simulink model "FKtest2"  (Simulink 6.6)
settings: Solver=ode4  StartTime=0.0  StopTime=400  FixedStep=0.05  RelTol=1e-3
values from neighbouring files (symbols this model uses):
  vessel =     [input.mat]    (also in supply.mat)
libraries: marine_gnc x10, simulink x1
(part 1 of 2)
settings Model: Creator=Thor  LastModifiedBy=Thor

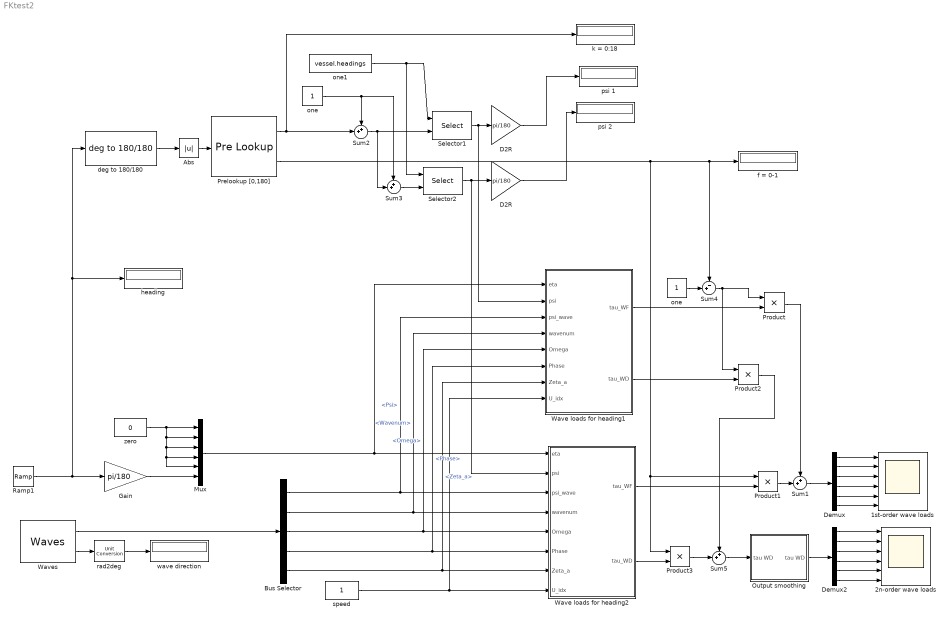
== system FKtest2 ==
  "1st-order wave loads " : Scope  NumInputPorts=6
      settings: TimeRange=100  YMin=-4e+006~-7.5e+006~-2e+007~-1e+007~-3.5e+008~-7.5e+007  YMax=4e+006~1e+007~2e+007~1e+007~3e+008~7.5e+007
  2n-order wave loads : Scope  NumInputPorts=6
      settings: TimeRange=400  YMin=-50000~-250000~-1~-1~-1~-900000  YMax=20000~25000~1~1~1~100000
  Abs : Abs  SaturateOnIntegerOverflow=on
  Bus Selector : BusSelector  OutputSignals=Psi,Wavenum,Omega,Phase,Zeta_a
  D2R : Gain  Gain=pi/180
  "D2R " : Gain  Gain=pi/180
  Demux : Demux  Outputs=6
  Demux2 : Demux  Outputs=6
  Gain : Gain  Gain=pi/180
  Mux : Mux  Inputs=6
  Output smoothing : Subsystem
  Prelookup [0,180] : PreLookup  BreakpointsData=[0:10:180]  IndexSearchMethod=Evenly spaced points  BeginIndexSearchUsingPreviousIndexResult=on
  Product{,1..3} (4 alike) : Product  RndMeth=Zero
  Ramp1 : simulink/Sources/Ramp  SystemSampleTime=-1  slope=1  start=0  X0=0
  Selector1 : Selector  IndexOptions=Index vector (port)  Indices=[1 3]  OutputSizes=1
  Selector2 : Selector  IndexOptions=Index vector (port)  Indices=[1 3]  OutputSizes=1
  Sum{1..3,5} (4 alike) : Sum  Inputs=++|
  Sum4 : Sum  Inputs=-+|
  Wave loads for heading1 : Subsystem  AncestorBlock=marine_gnc/Models/Environmental Loads/Force RAO  mask(Force RAO){ForceRAO_Freq=vessel.forceRAO.w, WD_Freq=vessel.driftfrc.w, RAO_Dir=vessel.headings, RAO_Vel=vessel.velocities, ForceRAO_Amp=vessel.forceRAO.amp, ForceRAO_Phase=vessel.forceRAO.phase, WD_Amp=vessel.driftfrc.amp, RAO_add_omega_0=off, RAO_add_omega_inf=off, RAO_speed_backlash_flag=off, RAO_speed_back=1}
      mask prompts: ForceRAO_Freq "Vector of frequencies ForceRAO_Freq (rad/s)"; WD_Freq "Vector of frequencies WD_Freq (rad/s)"; RAO_Dir "Vector of directions RAO_Dir (rad)"; RAO_Vel "Vector of velocities RAO_Vel (m/s)"; ForceRAO_Amp "6DOF Cell array with tables of Amplitudes ForceRAO_Amp"; ForceRAO_Phase "6DOF Cell array with tables of Phases ForceRAO_Phase (rad)"; WD_Amp "6DOF Cell array with tables of Amplitudes WD_Amp"; RAO_add_omega_0 "Add asymptotic RAO values for omega = 0"; RAO_add_omega_inf "Add asymptotic RAO values for omega = inf"; RAO_speed_backlash_flag "Speed lookup backlash (avoid rapid speed data switching)"; RAO_speed_back "Speed backlash widht [m/s]"
      mask help:
      | Calculate the 6 degrees-of-freedom (DOF) wave-frequency excitation forces Tau_WF for a vessel from its Force Response Amplitude Operators (Force RAOs) and a sea state defined by a set of harmonic waves. The block takes the "Waves" bus from the MSS Waves block as input, as well as the vessel low-frequency (LF) motion in terms of the generalized position vector eta_LF and mean surge velocity U. See help for details.
      |
      | Copyright (C) NTNU 2005
      | Author: Oyvind N. Smogeli, 2005-05-03
      mask init:
      | % Add RAO values for zero frequency: use values for lowest given frequency
      | if RAO_add_omega_0 > 0
      | 	
      | 	if min(ForceRAO_Freq) > 0
      | 				
      | 		ForceRAO_Freq = [0 ForceRAO_Freq];
      | 		for dofno = 1:6
      | 			ForceRAO_Amp{dofno}   = [ForceRAO_Amp{dofno}(1,:,:);   ForceRAO_Amp{dofno}];
      | 			ForceRAO_Phase{dofno} = [ForceRAO_Phase{dofno}(1,:,:); ForceRAO_Phase{dofno}];
      |         end
      | 
      |     end
      |     
      | 	if min(WD_Freq) > 0
      |         
      | 		WD_Freq = [0 WD_Freq];
      | 		for dofno = 1:3
      | 			WD_Amp{dofno} = [WD_Amp{dofno}(1,:,:); WD_Amp{dofno}];
      | 		end        
      |         
      | 	end
      | 	
      | end
      | 
      | % Add RAO values for high frequency: use values for highest given frequency
      | maxfreq = 100;
      | if RAO_add_omega_inf > 0
      | 
      | 	if max(ForceRAO_Freq) < maxfreq
      | 			
      | 		newfreq = 2*max(ForceRAO_Freq) - ForceRAO_Freq(length(ForceRAO_Freq)-1);
      | 		
      | 		ForceRAO_Freq = [ForceRAO_Freq newfreq maxfreq];
      | 		for dofno = 1:6
      | 			ForceRAO_Amp{dofno}   = [ForceRAO_Amp{dofno};   zeros(2, length(RAO_Dir), 10)];
      | 			ForceRAO_Phase{dofno} = [ForceRAO_Phase{dofno}; zeros(2, length(RAO_Dir), 10)];
      | 		end
      | 		
      |     end
      | 
      | 	if max(WD_Freq) < maxfreq
      | 			
      | 		newfreq = 2*max(WD_Freq) - WD_Freq(length(WD_Freq)-1);
      | 		
      | 		WD_Freq = [WD_Freq newfreq maxfreq];
      | 		for dofno = 1:3
      | 			WD_Amp{dofno} = [WD_Amp{dofno}; zeros(2, length(RAO_Dir), 10)];
      | 		end
      | 		
      |     end
      |     
      | end
      mask Help:
      | <b>Part of the Marine Systems Simulator: MSS</b><br>
      | <br>
      | Calculate the 6 degrees-of-freedom (DOF) wave-frequency excitation forces Tau_WF
      | for a vessel from its Force Response Amplitude Operators (Force RAOs) and a sea
      | state defined by a set of harmonic waves. The block takes the &quot;Waves&quot; bus from
      | the MSS Waves block as input, as well as the vessel low-frequency (LF) motion in
      | terms of the generalized position vector eta_LF and mean surge velocity U.<p>The Force RAOs are defined in terms of a
      | vector of frequencies (RAO_Freq), a vector of directions (RAO_Dir), a vector of
      | velocities (RAO_Dir), a 6DOF cell array of 3D matrices with amplitudes
      | (RAO_Amp), and a 6DOF cell array of 3D matrices with phases (RAO_Phase), which
      | are all input in the block mask. The first dimension of the 3D matrices
      | corresponds to the frequencies, the second to the directions, and the third to
      | the velocities, such that e.g. the amplitude amp in heave (DOF #3) for frequency
      | number n_f, direction number n_d and velocity number n_v can be found from a =
      | RAO_Amp{3}(n_f, n_d, n_v).</p>
      | <p><b>Inputs:</b></p>
      | <p>Waves:&nbsp;&nbsp;&nbsp;&nbsp;&nbsp;&nbsp;&nbsp;&nbsp;&nbsp;&nbsp;&nbsp; Bus
      | containing the following signals<br>
      | &nbsp;&nbsp;&nbsp; Zeta_a:&nbsp;&nbsp;&nbsp;&nbsp;&nbsp;&nbsp;&nbsp; Vector of harmonic wave amplitudes [m]<br>
      | &nbsp;&nbsp;&nbsp; Omega:&nbsp;&nbsp;&nbsp;&nbsp;&nbsp;&nbsp; Vector of harmonic wave frequencies [rad/s]<br>
      | &nbsp;&nbsp;&nbsp; Phase:&nbsp;&nbsp;&nbsp;&nbsp;&nbsp;&nbsp;&nbsp;&nbsp; Vector of harmonic wave phases (random) [rad]<br>
      | &nbsp;&nbsp;&nbsp; Wavenum:&nbsp;&nbsp;&nbsp; Vector of harmonic wave numbers [1/m]<br>
      | &nbsp;&nbsp;&nbsp; Psi:&nbsp;&nbsp;&nbsp;&nbsp;&nbsp;&nbsp;&nbsp;&nbsp;&nbsp;&nbsp;&nbsp;&nbsp;&nbsp; Vector of harmonic wave directions [rad]</p>
      | <p>eta_LF:&nbsp;&nbsp;&nbsp;&nbsp;&nbsp;&nbsp;&nbsp;&nbsp;&nbsp;&nbsp;&nbsp;
      | Generalized 6DOF n-frame low-frequency position vector [x (m), y (m), z (m),
      | theta (rad), phi (rad), psi (rad)]<br>
      | U:&nbsp;&nbsp;&nbsp;&nbsp;&nbsp;&nbsp;&nbsp;&nbsp;&nbsp;&nbsp;&nbsp;&nbsp;&nbsp;&nbsp;&nbsp;&nbsp;&nbsp;&nbsp;&nbsp;
      | Low-frequency (mean) surge velocity&nbsp; [m/s]</p>
      | <p><b>Outputs:</b></p>
      | <p>tau_WF:&nbsp;&nbsp;&nbsp;&nbsp;&nbsp;&nbsp;&nbsp;&nbsp;&nbsp; Generalized
      | 6DOF h-frame force vector [X (N), Y (N), Z (N), K (Nm), M (Nm), N (Nm)]</p>
      | <p><b>Model validity:</b></p>
      | <p>The validity of the block is dependent on the validity of the given
      | RAO data set.</p>
      | <p>A proper RAO to be used with this block should contain at least 1 velocity, 5
      | directions (e.g. 0, 45, 90, 135 and 180 degrees) and 10-20 frequencies, for all
      | 6 DOF (surge, sway, heave, roll, pitch, yaw).</p>
      | <p>The block performs linear interpolation in frequencies and directions, and
      | uses the data set for the velocity closest to the input velocity (i.e. 'nearest'
      | interpolation in velocity). If the block recieves an input wave frequency or relative
      | wave direction outside the span of the data vectors RAO_Freq or RAO_Dir
      | respectively, the simulation stops and an error is returned. This means that a well-defined
      | RAO must contain data for both 0 and 180 degrees, and for frequencies covering
      | the desired range of wave frequencies. If desired, asymptotic values can be
      | automatically added for zero and infinity frequency to avoid runtime errors if
      | the wave freqeuncy exceeds the values in RAO_Freq (see checkboxes in the mask). </p>
      | <p>IMPORTANT NOTE: The RAO theory upon which this block is based is in reality
      | only valid when the vessel low-frequency (h-frame) motion is a constant surge
      | velocity only, and the vessel is performing wave-frequency oscillations about
      | the steadily translating h-frame.This means that the outputs from the block when
      | manoeuvering -- i.e. changing the surge velocity and/or yaw angle -- must be
      | interpreted with some care. A jump in the output must be expected when changing
      | between two velocity data sets, and frequency warping expected when changing the
      | yaw angle (due to interpolation in the phase). It is therefore recommended to
      | use backlash on the input velocity to avoid transient switching, and a quantized
      | yaw angle with backlash. The latter will lead to jump in the ouput when the yaw
      | angle changes from one quantized value to another, but will give better results
      | when keeping within one quantizer interval. The quantized yaw angle with
      | backlash and velocity with backlash are available as options via checkboxes in
      | the mask. If either of these are activated, proper values for the yaw
      | quantization interval, yaw backlash width, and the the speed backlash width
      | respectively must be set. Typical values could be a yaw quantization interval of
      | 5 degrees, yaw backlash width of 1/4-1/5 of the quantization interval, and speed
      | backlash width of 1 m/s. To avoid the most rapid transients when switching
      | between data sets, output smoothing is available as an option in the mask. If
      | this is enabled, the output during a transent is rate limited according to the
      | fastest recorded signal rate during normal operation.</p>
      | <p><b>Example mask input:</b></p><p>
      | As an example, the format of the mask input for 2 velocities, 3 directions and 5
      | frequencies is as follows:<p>RAO_Freq = [f1 f2 f3 f4 f5]<br>
      | RAO_Dir = [d1 d2 d3]<br>
      | RAO_Vel = [v1 v2]<p>Surge:<br>
      | RAO_Amp{1}(:,:,1)&nbsp; = [a1_111 a1_121 a1_131; a1_211 a1_221 a1_231; a1_311
      | a1_321 a1_331; a1_411 a1_421 a1_431; a1_511 a1_521 a1_531]<br>
      | RAO_Amp{1}(:,:,2)&nbsp; = [a1_112 a1_122 a1_132; a1_212 a1_222 a1_232; a1_312
      | a1_322 a1_332; a1_412 a1_422 a1_432; a1_512 a1_522 a1_532]<br>
      | RAO_Phase{1}(:,:,1) = [p1_111 p1_121 p1_131; p1_211 p1_221 p1_231; p1_311 p1_321
      | p1_331; p1_411 p1_421 p1_431; p1_511 p1_521 p1_531]<br>
      | RAO_Phase{1}(:,:,2) = [p1_112 p1_122 p1_132; p1_212 p1_222 p1_232; p1_312 p1_322
      | p1_332; p1_412 p1_422 p1_432; p1_512 p1_522 p1_532]<p>Sway:<br>
      | RAO_Amp{2}(:,:,1)&nbsp; = [a2_111 a2_121 a2_131; a2_211 a2_221 a2_231; a2_311
      | a2_321 a2_331; a2_411 a2_421 a2_431; a2_511 a2_521 a2_531]<br>
      | RAO_Amp{2}(:,:,2)&nbsp; = [a2_112 a2_122 a2_132; a2_212 a2_222 a2_232; a2_312
      | a2_322 a2_332; a2_412 a2_422 a2_432; a2_512 a2_522 a2_532]<br>
      | RAO_Phase{2}(:,:,1) = [p2_111 p2_121 p2_131; p2_211 p2_221 p2_231; p2_311 p2_321
      | p2_331; p2_411 p2_421 p2_431; p2_511 p2_521 p2_531]<br>
      | RAO_Phase{2}(:,:,2) = [p2_112 p2_122 p2_132; p2_212 p2_222 p2_232; p2_312 p2_322
      | p2_332; p2_412 p2_422 p2_432; p2_512 p2_522 p2_532]<p>...<p>Yaw:<br>
      | RAO_Amp{6}(:,:,1)&nbsp; = [a6_111 a6_121 a6_131; a6_211 a6_221 a6_231; a6_311
      | a6_321 a6_331; a6_411 a6_421 a6_431; a6_511 a6_521 a6_531]<br>
      | RAO_Amp{6}(:,:,2)&nbsp; = [a6_112 a6_122 a6_132; a6_212 a6_222 a6_232; a6_312
      | a6_322 a6_332; a6_412 a6_422 a6_432; a6_512 a6_522 a6_532]<br>
      | RAO_Phase{6}(:,:,1) = [p6_111 p6_121 p6_131; p6_211 p6_221 p6_231; p6_311 p6_321
      | p6_331; p6_411 p6_421 p6_431; p6_511 p6_521 p6_531]<br>
      | RAO_Phase{6}(:,:,2) = [p6_112 p6_122 p6_132; p6_212 p6_222 p6_232; p6_312 p6_322
      | p6_332; p6_412 p6_422 p6_432; p6_512 p6_522 p6_532]<p>where now for example the
      | amplitude and phase in sway (DOF 2) for frequency f5, direction d3 and velocity
      | v1 are given by RAO_Amp{2}(5,3,1) = a2_531 and RAO_Phase{2}(5,3,1) = p2_531.<p>
      | <b>Copyright (C) NTNU 2005</b></p>
      | <p><b>Author:</b> Oyvind N. Smogeli, 2005-05-03</p>
  Wave loads for heading2 : Subsystem  AncestorBlock=marine_gnc/Models/Environmental Loads/Force RAO  mask(Force RAO){ForceRAO_Freq=vessel.forceRAO.w, WD_Freq=vessel.driftfrc.w, RAO_Dir=vessel.headings, RAO_Vel=vessel.velocities, ForceRAO_Amp=vessel.forceRAO.amp, ForceRAO_Phase=vessel.forceRAO.phase, WD_Amp=vessel.driftfrc.amp, RAO_add_omega_0=on, RAO_add_omega_inf=on, RAO_speed_backlash_flag=off, RAO_speed_back=1}
      mask prompts: ForceRAO_Freq "Vector of frequencies ForceRAO_Freq (rad/s)"; WD_Freq "Vector of frequencies WD_Freq (rad/s)"; RAO_Dir "Vector of directions RAO_Dir (rad)"; RAO_Vel "Vector of velocities RAO_Vel (m/s)"; ForceRAO_Amp "6DOF Cell array with tables of Amplitudes ForceRAO_Amp"; ForceRAO_Phase "6DOF Cell array with tables of Phases ForceRAO_Phase (rad)"; WD_Amp "6DOF Cell array with tables of Amplitudes WD_Amp"; RAO_add_omega_0 "Add asymptotic RAO values for omega = 0"; RAO_add_omega_inf "Add asymptotic RAO values for omega = inf"; RAO_speed_backlash_flag "Speed lookup backlash (avoid rapid speed data switching)"; RAO_speed_back "Speed backlash widht [m/s]"
      mask help:
      | Calculate the 6 degrees-of-freedom (DOF) wave-frequency excitation forces Tau_WF for a vessel from its Force Response Amplitude Operators (Force RAOs) and a sea state defined by a set of harmonic waves. The block takes the "Waves" bus from the MSS Waves block as input, as well as the vessel low-frequency (LF) motion in terms of the generalized position vector eta_LF and mean surge velocity U. See help for details.
      |
      | Copyright (C) NTNU 2005
      | Author: Oyvind N. Smogeli, 2005-05-03
      mask init: same as FKtest2/Wave loads for heading1
      mask Help:
      | <b>Part of the Marine Systems Simulator: MSS</b><br>
      | <br>
      | Calculate the 6 degrees-of-freedom (DOF) wave-frequency excitation forces Tau_WF
      | for a vessel from its Force Response Amplitude Operators (Force RAOs) and a sea
      | state defined by a set of harmonic waves. The block takes the &quot;Waves&quot; bus from
      | the MSS Waves block as input, as well as the vessel low-frequency (LF) motion in
      | terms of the generalized position vector eta_LF and mean surge velocity U.<p>The Force RAOs are defined in terms of a
      | vector of frequencies (RAO_Freq), a vector of directions (RAO_Dir), a vector of
      | velocities (RAO_Dir), a 6DOF cell array of 3D matrices with amplitudes
      | (RAO_Amp), and a 6DOF cell array of 3D matrices with phases (RAO_Phase), which
      | are all input in the block mask. The first dimension of the 3D matrices
      | corresponds to the frequencies, the second to the directions, and the third to
      | the velocities, such that e.g. the amplitude amp in heave (DOF #3) for frequency
      | number n_f, direction number n_d and velocity number n_v can be found from a =
      | RAO_Amp{3}(n_f, n_d, n_v).</p>
      | <p><b>Inputs:</b></p>
      | <p>Waves:&nbsp;&nbsp;&nbsp;&nbsp;&nbsp;&nbsp;&nbsp;&nbsp;&nbsp;&nbsp;&nbsp; Bus
      | containing the following signals<br>
      | &nbsp;&nbsp;&nbsp; Zeta_a:&nbsp;&nbsp;&nbsp;&nbsp;&nbsp;&nbsp;&nbsp; Vector of harmonic wave amplitudes [m]<br>
      | &nbsp;&nbsp;&nbsp; Omega:&nbsp;&nbsp;&nbsp;&nbsp;&nbsp;&nbsp; Vector of harmonic wave frequencies [rad/s]<br>
      | &nbsp;&nbsp;&nbsp; Phase:&nbsp;&nbsp;&nbsp;&nbsp;&nbsp;&nbsp;&nbsp;&nbsp; Vector of harmonic wave phases (random) [rad]<br>
      | &nbsp;&nbsp;&nbsp; Wavenum:&nbsp;&nbsp;&nbsp; Vector of harmonic wave numbers [1/m]<br>
      | &nbsp;&nbsp;&nbsp; Psi:&nbsp;&nbsp;&nbsp;&nbsp;&nbsp;&nbsp;&nbsp;&nbsp;&nbsp;&nbsp;&nbsp;&nbsp;&nbsp; Vector of harmonic wave directions [rad]</p>
      | <p>eta_LF:&nbsp;&nbsp;&nbsp;&nbsp;&nbsp;&nbsp;&nbsp;&nbsp;&nbsp;&nbsp;&nbsp;
      | Generalized 6DOF n-frame low-frequency position vector [x (m), y (m), z (m),
      | theta (rad), phi (rad), psi (rad)]<br>
      | U:&nbsp;&nbsp;&nbsp;&nbsp;&nbsp;&nbsp;&nbsp;&nbsp;&nbsp;&nbsp;&nbsp;&nbsp;&nbsp;&nbsp;&nbsp;&nbsp;&nbsp;&nbsp;&nbsp;
      | Low-frequency (mean) surge velocity&nbsp; [m/s]</p>
      | <p><b>Outputs:</b></p>
      | <p>tau_WF:&nbsp;&nbsp;&nbsp;&nbsp;&nbsp;&nbsp;&nbsp;&nbsp;&nbsp; Generalized
      | 6DOF h-frame force vector [X (N), Y (N), Z (N), K (Nm), M (Nm), N (Nm)]</p>
      | <p><b>Model validity:</b></p>
      | <p>The validity of the block is dependent on the validity of the given
      | RAO data set.</p>
      | <p>A proper RAO to be used with this block should contain at least 1 velocity, 5
      | directions (e.g. 0, 45, 90, 135 and 180 degrees) and 10-20 frequencies, for all
      | 6 DOF (surge, sway, heave, roll, pitch, yaw).</p>
      | <p>The block performs linear interpolation in frequencies and directions, and
      | uses the data set for the velocity closest to the input velocity (i.e. 'nearest'
      | interpolation in velocity). If the block recieves an input wave frequency or relative
      | wave direction outside the span of the data vectors RAO_Freq or RAO_Dir
      | respectively, the simulation stops and an error is returned. This means that a well-defined
      | RAO must contain data for both 0 and 180 degrees, and for frequencies covering
      | the desired range of wave frequencies. If desired, asymptotic values can be
      | automatically added for zero and infinity frequency to avoid runtime errors if
      | the wave freqeuncy exceeds the values in RAO_Freq (see checkboxes in the mask). </p>
      | <p>IMPORTANT NOTE: The RAO theory upon which this block is based is in reality
      | only valid when the vessel low-frequency (h-frame) motion is a constant surge
      | velocity only, and the vessel is performing wave-frequency oscillations about
      | the steadily translating h-frame.This means that the outputs from the block when
      | manoeuvering -- i.e. changing the surge velocity and/or yaw angle -- must be
      | interpreted with some care. A jump in the output must be expected when changing
      | between two velocity data sets, and frequency warping expected when changing the
      | yaw angle (due to interpolation in the phase). It is therefore recommended to
      | use backlash on the input velocity to avoid transient switching, and a quantized
      | yaw angle with backlash. The latter will lead to jump in the ouput when the yaw
      | angle changes from one quantized value to another, but will give better results
      | when keeping within one quantizer interval. The quantized yaw angle with
      | backlash and velocity with backlash are available as options via checkboxes in
      | the mask. If either of these are activated, proper values for the yaw
      | quantization interval, yaw backlash width, and the the speed backlash width
      | respectively must be set. Typical values could be a yaw quantization interval of
      | 5 degrees, yaw backlash width of 1/4-1/5 of the quantization interval, and speed
      | backlash width of 1 m/s. To avoid the most rapid transients when switching
      | between data sets, output smoothing is available as an option in the mask. If
      | this is enabled, the output during a transent is rate limited according to the
      | fastest recorded signal rate during normal operation.</p>
      | <p><b>Example mask input:</b></p><p>
      | As an example, the format of the mask input for 2 velocities, 3 directions and 5
      | frequencies is as follows:<p>RAO_Freq = [f1 f2 f3 f4 f5]<br>
      | RAO_Dir = [d1 d2 d3]<br>
      | RAO_Vel = [v1 v2]<p>Surge:<br>
      | RAO_Amp{1}(:,:,1)&nbsp; = [a1_111 a1_121 a1_131; a1_211 a1_221 a1_231; a1_311
      | a1_321 a1_331; a1_411 a1_421 a1_431; a1_511 a1_521 a1_531]<br>
      | RAO_Amp{1}(:,:,2)&nbsp; = [a1_112 a1_122 a1_132; a1_212 a1_222 a1_232; a1_312
      | a1_322 a1_332; a1_412 a1_422 a1_432; a1_512 a1_522 a1_532]<br>
      | RAO_Phase{1}(:,:,1) = [p1_111 p1_121 p1_131; p1_211 p1_221 p1_231; p1_311 p1_321
      | p1_331; p1_411 p1_421 p1_431; p1_511 p1_521 p1_531]<br>
      | RAO_Phase{1}(:,:,2) = [p1_112 p1_122 p1_132; p1_212 p1_222 p1_232; p1_312 p1_322
      | p1_332; p1_412 p1_422 p1_432; p1_512 p1_522 p1_532]<p>Sway:<br>
      | RAO_Amp{2}(:,:,1)&nbsp; = [a2_111 a2_121 a2_131; a2_211 a2_221 a2_231; a2_311
      | a2_321 a2_331; a2_411 a2_421 a2_431; a2_511 a2_521 a2_531]<br>
      | RAO_Amp{2}(:,:,2)&nbsp; = [a2_112 a2_122 a2_132; a2_212 a2_222 a2_232; a2_312
      | a2_322 a2_332; a2_412 a2_422 a2_432; a2_512 a2_522 a2_532]<br>
      | RAO_Phase{2}(:,:,1) = [p2_111 p2_121 p2_131; p2_211 p2_221 p2_231; p2_311 p2_321
      | p2_331; p2_411 p2_421 p2_431; p2_511 p2_521 p2_531]<br>
      | RAO_Phase{2}(:,:,2) = [p2_112 p2_122 p2_132; p2_212 p2_222 p2_232; p2_312 p2_322
      | p2_332; p2_412 p2_422 p2_432; p2_512 p2_522 p2_532]<p>...<p>Yaw:<br>
      | RAO_Amp{6}(:,:,1)&nbsp; = [a6_111 a6_121 a6_131; a6_211 a6_221 a6_231; a6_311
      | a6_321 a6_331; a6_411 a6_421 a6_431; a6_511 a6_521 a6_531]<br>
      | RAO_Amp{6}(:,:,2)&nbsp; = [a6_112 a6_122 a6_132; a6_212 a6_222 a6_232; a6_312
      | a6_322 a6_332; a6_412 a6_422 a6_432; a6_512 a6_522 a6_532]<br>
      | RAO_Phase{6}(:,:,1) = [p6_111 p6_121 p6_131; p6_211 p6_221 p6_231; p6_311 p6_321
      | p6_331; p6_411 p6_421 p6_431; p6_511 p6_521 p6_531]<br>
      | RAO_Phase{6}(:,:,2) = [p6_112 p6_122 p6_132; p6_212 p6_222 p6_232; p6_312 p6_322
      | p6_332; p6_412 p6_422 p6_432; p6_512 p6_522 p6_532]<p>where now for example the
      | amplitude and phase in sway (DOF 2) for frequency f5, direction d3 and velocity
      | v1 are given by RAO_Amp{2}(5,3,1) = a2_531 and RAO_Phase{2}(5,3,1) = p2_531.<p>
      | <b>Copyright (C) NTNU 2005</b></p>
      | <p><b>Author:</b> Oyvind N. Smogeli, 2005-05-03</p>
  Waves : marine_gnc/Environment/Waves/Waves  SystemSampleTime=-1  spectrum_type=ITTC  disp_flag=off  plot_spectrum=off  plot_realization=off  hs=5  omega_peak=-1  psi_mean=0/(180/pi)  gamma=-1  spread=2  depth=inf  nfreq=20  ndir=10  energylim=0.005  freq_cutoff=3  dir_cutoff=0  rand_seed=0  rand_freq=on  rand_dir=on  Zeta_a=0  Omega=0  Phase=0  Wavenum=0  Psi=0
  deg to 180/180 : marine_gnc/Utilities/Math Operations/deg to 180//180  SystemSampleTime=-1
  f = 0-1 : Display
  heading : Display
  k = 0:18 : Display
  one : Constant
  "one " : Constant
  one1 : Constant  Value=vessel.headings
  psi 1 : Display
  psi 2 : Display
  rad2deg : marine_gnc/Utilities/Math Operations/Unit Conversion  SystemSampleTime=-1  in=rad2deg
  speed : Constant
  wave direction : Display
  zero : Constant  Value=0
  wires:
  speed/1 -> Wave loads for heading1/8(U_idx), Wave loads for heading2/8(U_idx)
  Ramp1/1 -> Gain/1, heading/1, deg to 180/180/1
  Waves/2 -> rad2deg/1
  rad2deg/1 -> wave direction/1
  Demux/1 -> "1st-order wave loads "/1
  Demux/2 -> "1st-order wave loads "/2
  Demux/3 -> "1st-order wave loads "/3
  Demux/4 -> "1st-order wave loads "/4
  Demux/5 -> "1st-order wave loads "/5
  Demux/6 -> "1st-order wave loads "/6
  Wave loads for heading2/1(tau_WF) -> Product1/2
  Demux2/1 -> 2n-order wave loads/1
  Demux2/2 -> 2n-order wave loads/2
  Demux2/3 -> 2n-order wave loads/3
  Demux2/4 -> 2n-order wave loads/4
  Demux2/5 -> 2n-order wave loads/5
  Demux2/6 -> 2n-order wave loads/6
  Wave loads for heading2/2(tau_WD) -> Product3/2
  Mux/1 -> Wave loads for heading1/1(eta), Wave loads for heading2/1(eta)
  zero/1 -> Mux/1, Mux/2, Mux/3, Mux/4, Mux/5
  Bus Selector/1 -> Wave loads for heading1/3(psi_wave), Wave loads for heading2/3(psi_wave)  "<Psi>"
  Waves/1 -> Bus Selector/1
  Bus Selector/2 -> Wave loads for heading1/4(wavenum), Wave loads for heading2/4(wavenum)  "<Wavenum>"
  Bus Selector/3 -> Wave loads for heading1/5(Omega), Wave loads for heading2/5(Omega)  "<Omega>"
  Bus Selector/4 -> Wave loads for heading1/6(Phase), Wave loads for heading2/6(Phase)  "<Phase>"
  Bus Selector/5 -> Wave loads for heading1/7(Zeta_a), Wave loads for heading2/7(Zeta_a)  "<Zeta_a>"
  Gain/1 -> Mux/6
  Sum1/1 -> Demux/1
  Wave loads for heading1/1(tau_WF) -> Product/2
  Product/1 -> Sum1/1
  Product1/1 -> Sum1/2
  "one "/1 -> Sum4/2
  Sum4/1 -> Product/1, Product2/1
  Sum5/1 -> Output smoothing/1(tau WD)
  Wave loads for heading1/2(tau_WD) -> Product2/2
  Product3/1 -> Sum5/2
  Product2/1 -> Sum5/1
  Prelookup [0,180]/1 -> k = 0:18/1, Sum2/2
  one/1 -> Sum2/1, Sum3/1
  deg to 180/180/1 -> Abs/1
  Abs/1 -> Prelookup [0,180]/1
  Prelookup [0,180]/2 -> Product3/1, Product1/1, Sum4/1, f = 0-1/1
  Sum2/1 -> Sum3/2, Selector1/2
  one1/1 -> Selector1/1, Selector2/1
  Sum3/1 -> Selector2/2
  Selector1/1 -> D2R/1, Wave loads for heading1/2(psi)
  Selector2/1 -> "D2R "/1, Wave loads for heading2/2(psi)
  "D2R "/1 -> psi 2/1
  D2R/1 -> psi 1/1
  Output smoothing/1("tau WD ") -> Demux2/1

== system FKtest2/Output smoothing ==
  tau WD : Inport
  2nd order time constant 1 : marine_gnc/Utilities/Dynamics/2nd order time constant  SystemSampleTime=-1  T=5
  2nd order time constant 2 : marine_gnc/Utilities/Dynamics/2nd order time constant  SystemSampleTime=-1  T=5
  2nd order time constant 6 : marine_gnc/Utilities/Dynamics/2nd order time constant  SystemSampleTime=-1  T=5
  Demux : Demux  Outputs=6
  Mux : Mux  Inputs=6
  "tau WD " : Outport
  wires:
  Demux/1 -> 2nd order time constant 1/1
  Demux/2 -> 2nd order time constant 2/1
  Demux/3 -> Mux/3
  Demux/4 -> Mux/4
  Demux/5 -> Mux/5
  Demux/6 -> 2nd order time constant 6/1
  tau WD/1 -> Demux/1
  2nd order time constant 1/1 -> Mux/1
  2nd order time constant 2/1 -> Mux/2
  2nd order time constant 6/1 -> Mux/6
  Mux/1 -> "tau WD "/1

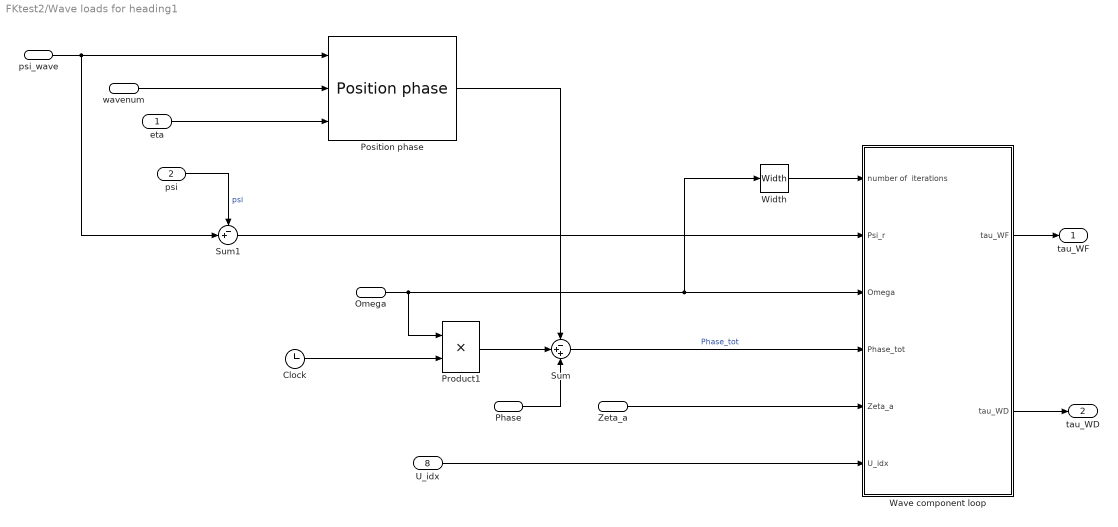
== system FKtest2/Wave loads for heading1 ==
  eta : Inport
  psi : Inport  Port=2
  psi_wave : Inport  Port=3
  wavenum : Inport  Port=4
  Omega : Inport  Port=5
  Phase : Inport  Port=6
  Zeta_a : Inport  Port=7
  U_idx : Inport  Port=8
  Clock : Clock
      settings: Decimation=10
  Position phase : marine_gnc/Models/Environmental Loads/Utilities/Position phase  SystemSampleTime=-1
  Product1 : Product  Inputs=**  SaturateOnIntegerOverflow=on
  Sum : Sum  Inputs=-++  SaturateOnIntegerOverflow=on
  Sum1 : Sum  Inputs=-+|
  Wave component loop : Subsystem  TreatAsAtomicUnit=on
  Width : Width  DataType=int32
  tau_WF : Outport
  tau_WD : Outport  Port=2
  wires:
  Position phase/1 -> Sum/1
  Width/1 -> Wave component loop/1(number of  iterations)
  Sum/1 -> Wave component loop/4(Phase_tot)  "Phase_tot"
  Clock/1 -> Product1/2
  Product1/1 -> Sum/2
  Wave component loop/1(tau_WF) -> tau_WF/1
  eta/1 -> Position phase/3
  psi_wave/1 -> Position phase/1, Sum1/2
  wavenum/1 -> Position phase/2
  Omega/1 -> Product1/1, Wave component loop/3(Omega), Width/1
  Phase/1 -> Sum/3
  Zeta_a/1 -> Wave component loop/5(Zeta_a)
  Sum1/1 -> Wave component loop/2(Psi_r)
  Wave component loop/2(tau_WD) -> tau_WD/1
  U_idx/1 -> Wave component loop/6(U_idx)
  psi/1 -> Sum1/1  "psi"

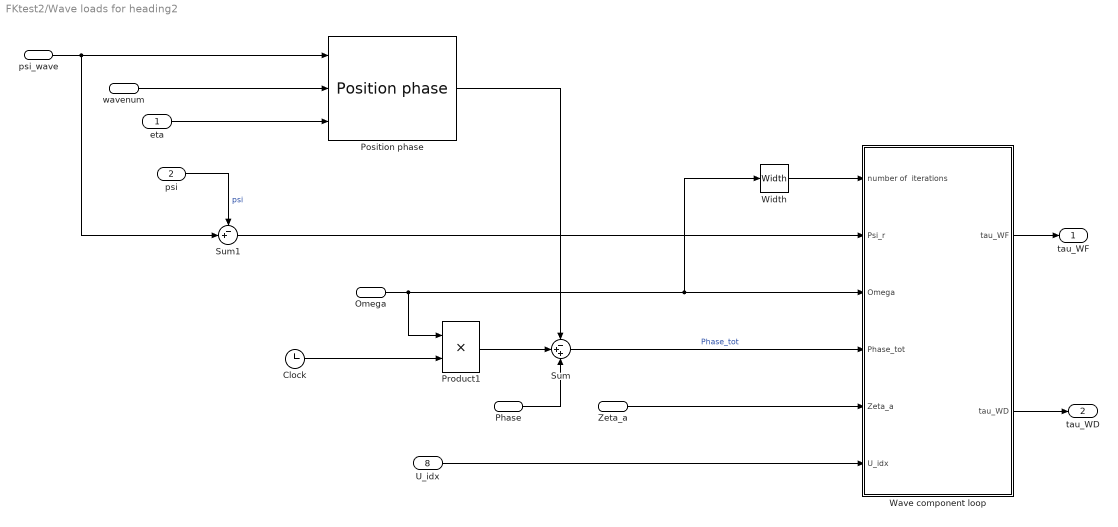
== system FKtest2/Wave loads for heading2 ==
  eta : Inport
  psi : Inport  Port=2
  psi_wave : Inport  Port=3
  wavenum : Inport  Port=4
  Omega : Inport  Port=5
  Phase : Inport  Port=6
  Zeta_a : Inport  Port=7
  U_idx : Inport  Port=8
  Clock : Clock
      settings: Decimation=10
  Position phase : marine_gnc/Models/Environmental Loads/Utilities/Position phase  SystemSampleTime=-1
  Product1 : Product  Inputs=**  SaturateOnIntegerOverflow=on
  Sum : Sum  Inputs=-++  SaturateOnIntegerOverflow=on
  Sum1 : Sum  Inputs=-+|
  Wave component loop : Subsystem  TreatAsAtomicUnit=on
  Width : Width  DataType=int32
  tau_WF : Outport
  tau_WD : Outport  Port=2
  wires:
  Position phase/1 -> Sum/1
  Width/1 -> Wave component loop/1(number of  iterations)
  Sum/1 -> Wave component loop/4(Phase_tot)  "Phase_tot"
  Clock/1 -> Product1/2
  Product1/1 -> Sum/2
  Wave component loop/1(tau_WF) -> tau_WF/1
  eta/1 -> Position phase/3
  psi_wave/1 -> Position phase/1, Sum1/2
  wavenum/1 -> Position phase/2
  Omega/1 -> Product1/1, Wave component loop/3(Omega), Width/1
  Phase/1 -> Sum/3
  Zeta_a/1 -> Wave component loop/5(Zeta_a)
  Sum1/1 -> Wave component loop/2(Psi_r)
  Wave component loop/2(tau_WD) -> tau_WD/1
  U_idx/1 -> Wave component loop/6(U_idx)
  psi/1 -> Sum1/1  "psi"

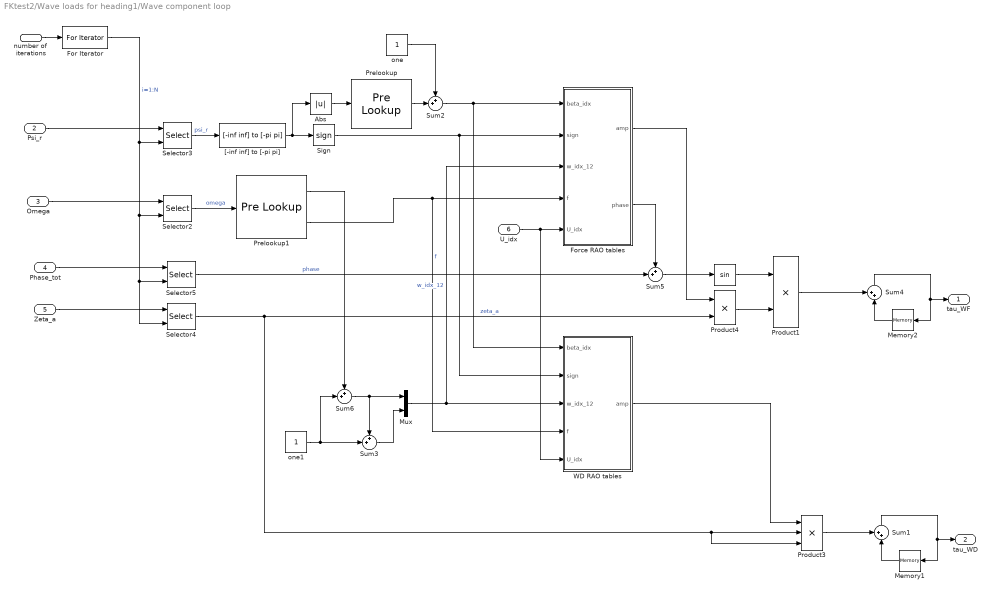
== system FKtest2/Wave loads for heading1/Wave component loop ==
  number of  iterations : Inport
  Psi_r : Inport  Port=2
  Omega : Inport  Port=3
  Phase_tot : Inport  Port=4
  Zeta_a : Inport  Port=5
  U_idx : Inport  Port=6
  "                " : Trigonometry
  Abs : Abs  SaturateOnIntegerOverflow=on
  For Iterator : ForIterator  ResetStates=reset  IterationSource=external  IterationVariableDataType=double
  Force RAO tables : Subsystem  AncestorBlock=marine_gnc/Models/Environmental Loads/Utilities/RAO tables  mask(RAO table lookup){RAO_Freq=ForceRAO_Freq, RAO_Dir=RAO_Dir, RAO_Vel=RAO_Vel, RAO_Amp=ForceRAO_Amp, RAO_Phase=ForceRAO_Phase}
      mask prompts: RAO_Freq "Vector of frequencies (rad/s)"; RAO_Dir "Vector of directions (rad)"; RAO_Vel "Vector of velocities (m/s)"; RAO_Amp "6DOF Cell array with tables of Amplitudes"; RAO_Phase "6DOF Cell array with tables of Phases (rad)"
      mask help:
      | Perform 3D table lookup in 6DOF RAO amplitudes and phases, using the relative wave heading psi_r, wave frequency omega and vessel velocity vel as inputs. See documentation of the Motion RAO block or Force RAO block for details. A warning is issued if the input is outside the range spanned by the RAOs.
      |
      | Copyright (C) NTNU 2005
      |
      | Author: Oyvind N. Smogeli, 2005-05-03
  Memory1 : Memory  Orientation=left  X0=[0 0 0 0 0 0]'  InheritSampleTime=on
  Memory2 : Memory  Orientation=left  X0=[0 0 0 0 0 0]'  InheritSampleTime=on
  Mux : Mux  Inputs=2
  Prelookup : PreLookup  BreakpointsData=vessel.headings  BeginIndexSearchUsingPreviousIndexResult=on  OutputOnlyTheIndex=on
  Prelookup1 : PreLookup  BreakpointsData=vessel.forceRAO.w  BeginIndexSearchUsingPreviousIndexResult=on  ProcessOutOfRangeInput=Linear extrapolation
  Product1 : Product  SaturateOnIntegerOverflow=on
  Product3 : Product  Inputs=3  SaturateOnIntegerOverflow=on
  Product4 : Product  SaturateOnIntegerOverflow=on
  Selector{2..5} (4 alike) : Selector  IndexOptions=Index vector (port)  Indices=[1 3]  OutputSizes=1
  Sign : Signum
  Sum1 : Sum  Orientation=up  Inputs=++|  SaturateOnIntegerOverflow=on
  Sum2 : Sum  Inputs=++|
  Sum3 : Sum  Inputs=++|
  Sum4 : Sum  Orientation=up  Inputs=++|  SaturateOnIntegerOverflow=on
  Sum5 : Sum  Inputs=++|  SaturateOnIntegerOverflow=on
  Sum6 : Sum  Inputs=++|
  WD RAO tables : Subsystem  AncestorBlock=marine_gnc/Models/Environmental Loads/Utilities/RAO tables  mask(RAO table lookup){RAO_Freq=ForceRAO_Freq, RAO_Dir=RAO_Dir, RAO_Vel=RAO_Vel, RAO_Amp=ForceRAO_Amp, RAO_Phase=ForceRAO_Phase}
      mask prompts: RAO_Freq "Vector of frequencies (rad/s)"; RAO_Dir "Vector of directions (rad)"; RAO_Vel "Vector of velocities (m/s)"; RAO_Amp "6DOF Cell array with tables of Amplitudes"; RAO_Phase "6DOF Cell array with tables of Phases (rad)"
      mask help:
      | Perform 3D table lookup in 6DOF RAO amplitudes and phases, using the relative wave heading psi_r, wave frequency omega and vessel velocity vel as inputs. See documentation of the Motion RAO block or Force RAO block for details. A warning is issued if the input is outside the range spanned by the RAOs.
      |
      | Copyright (C) NTNU 2005
      |
      | Author: Oyvind N. Smogeli, 2005-05-03
  "[-inf inf] to [-pi pi]" : marine_gnc/Utilities/Math Operations/[-inf inf] to [-pi pi]  SystemSampleTime=-1
  one : Constant
  one1 : Constant
  tau_WF : Outport
  tau_WD : Outport  Port=2
  wires:
  Selector4/1 -> Product4/2, Product3/2, Product3/3  "zeta_a"
  Sum5/1 -> "                "/1
  Zeta_a/1 -> Selector4/1
  Phase_tot/1 -> Selector5/1
  Force RAO tables/2(phase) -> Sum5/1
  Force RAO tables/1(amp) -> Product4/1
  U_idx/1 -> Force RAO tables/5(U_idx), WD RAO tables/5(U_idx)
  Psi_r/1 -> Selector3/1
  For Iterator/1 -> Selector3/2, Selector2/2, Selector5/2, Selector4/2  "i=1:N"
  Omega/1 -> Selector2/1
  number of  iterations/1 -> For Iterator/1
  Sum4/1 -> Memory2/1, tau_WF/1
  Memory2/1 -> Sum4/2
  Product1/1 -> Sum4/1
  Selector5/1 -> Sum5/2  "phase"
  Selector3/1 -> "[-inf inf] to [-pi pi]"/1  "psi_r"
  "                "/1 -> Product1/1
  Product4/1 -> Product1/2
  one/1 -> Sum2/1
  Sum2/1 -> Force RAO tables/1(beta_idx), WD RAO tables/1(beta_idx)
  Prelookup/1 -> Sum2/2
  Abs/1 -> Prelookup/1
  Sign/1 -> Force RAO tables/2(sign), WD RAO tables/2(sign)
  Sum1/1 -> Memory1/1, tau_WD/1
  Memory1/1 -> Sum1/2
  Product3/1 -> Sum1/1
  WD RAO tables/1(amp) -> Product3/1
  "[-inf inf] to [-pi pi]"/1 -> Abs/1, Sign/1
  Prelookup1/1 -> Sum6/1
  one1/1 -> Sum3/2, Sum6/2
  Sum3/1 -> Mux/2
  Sum6/1 -> Sum3/1, Mux/1
  Selector2/1 -> Prelookup1/1  "omega"
  Mux/1 -> Force RAO tables/3(w_idx_12), WD RAO tables/3(w_idx_12)  "w_idx_12"
  Prelookup1/2 -> Force RAO tables/4(f), WD RAO tables/4(f)  "f"

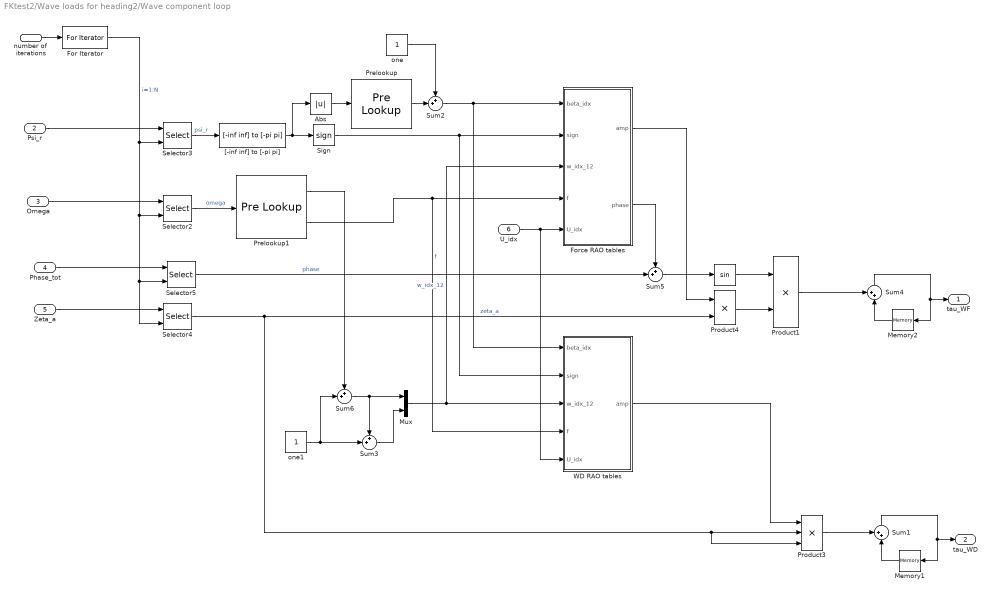
== system FKtest2/Wave loads for heading2/Wave component loop ==
  number of  iterations : Inport
  Psi_r : Inport  Port=2
  Omega : Inport  Port=3
  Phase_tot : Inport  Port=4
  Zeta_a : Inport  Port=5
  U_idx : Inport  Port=6
  "                " : Trigonometry
  Abs : Abs  SaturateOnIntegerOverflow=on
  For Iterator : ForIterator  ResetStates=reset  IterationSource=external  IterationVariableDataType=double
  Force RAO tables : Subsystem  AncestorBlock=marine_gnc/Models/Environmental Loads/Utilities/RAO tables  mask(RAO table lookup){RAO_Freq=ForceRAO_Freq, RAO_Dir=RAO_Dir, RAO_Vel=RAO_Vel, RAO_Amp=ForceRAO_Amp, RAO_Phase=ForceRAO_Phase}
      mask prompts: RAO_Freq "Vector of frequencies (rad/s)"; RAO_Dir "Vector of directions (rad)"; RAO_Vel "Vector of velocities (m/s)"; RAO_Amp "6DOF Cell array with tables of Amplitudes"; RAO_Phase "6DOF Cell array with tables of Phases (rad)"
      mask help:
      | Perform 3D table lookup in 6DOF RAO amplitudes and phases, using the relative wave heading psi_r, wave frequency omega and vessel velocity vel as inputs. See documentation of the Motion RAO block or Force RAO block for details. A warning is issued if the input is outside the range spanned by the RAOs.
      |
      | Copyright (C) NTNU 2005
      |
      | Author: Oyvind N. Smogeli, 2005-05-03
  Memory1 : Memory  Orientation=left  X0=[0 0 0 0 0 0]'  InheritSampleTime=on
  Memory2 : Memory  Orientation=left  X0=[0 0 0 0 0 0]'  InheritSampleTime=on
  Mux : Mux  Inputs=2
  Prelookup : PreLookup  BreakpointsData=vessel.headings  BeginIndexSearchUsingPreviousIndexResult=on  OutputOnlyTheIndex=on
  Prelookup1 : PreLookup  BreakpointsData=vessel.forceRAO.w  BeginIndexSearchUsingPreviousIndexResult=on  ProcessOutOfRangeInput=Linear extrapolation
  Product1 : Product  SaturateOnIntegerOverflow=on
  Product3 : Product  Inputs=3  SaturateOnIntegerOverflow=on
  Product4 : Product  SaturateOnIntegerOverflow=on
  Selector{2..5} (4 alike) : Selector  IndexOptions=Index vector (port)  Indices=[1 3]  OutputSizes=1
  Sign : Signum
  Sum1 : Sum  Orientation=up  Inputs=++|  SaturateOnIntegerOverflow=on
  Sum2 : Sum  Inputs=++|
  Sum3 : Sum  Inputs=++|
  Sum4 : Sum  Orientation=up  Inputs=++|  SaturateOnIntegerOverflow=on
  Sum5 : Sum  Inputs=++|  SaturateOnIntegerOverflow=on
  Sum6 : Sum  Inputs=++|
  WD RAO tables : Subsystem  AncestorBlock=marine_gnc/Models/Environmental Loads/Utilities/RAO tables  mask(RAO table lookup){RAO_Freq=ForceRAO_Freq, RAO_Dir=RAO_Dir, RAO_Vel=RAO_Vel, RAO_Amp=ForceRAO_Amp, RAO_Phase=ForceRAO_Phase}
      mask prompts: RAO_Freq "Vector of frequencies (rad/s)"; RAO_Dir "Vector of directions (rad)"; RAO_Vel "Vector of velocities (m/s)"; RAO_Amp "6DOF Cell array with tables of Amplitudes"; RAO_Phase "6DOF Cell array with tables of Phases (rad)"
      mask help:
      | Perform 3D table lookup in 6DOF RAO amplitudes and phases, using the relative wave heading psi_r, wave frequency omega and vessel velocity vel as inputs. See documentation of the Motion RAO block or Force RAO block for details. A warning is issued if the input is outside the range spanned by the RAOs.
      |
      | Copyright (C) NTNU 2005
      |
      | Author: Oyvind N. Smogeli, 2005-05-03
  "[-inf inf] to [-pi pi]" : marine_gnc/Utilities/Math Operations/[-inf inf] to [-pi pi]  SystemSampleTime=-1
  one : Constant
  one1 : Constant
  tau_WF : Outport
  tau_WD : Outport  Port=2
  wires:
  Selector4/1 -> Product4/2, Product3/2, Product3/3  "zeta_a"
  Sum5/1 -> "                "/1
  Zeta_a/1 -> Selector4/1
  Phase_tot/1 -> Selector5/1
  Force RAO tables/2(phase) -> Sum5/1
  Force RAO tables/1(amp) -> Product4/1
  U_idx/1 -> Force RAO tables/5(U_idx), WD RAO tables/5(U_idx)
  Psi_r/1 -> Selector3/1
  For Iterator/1 -> Selector3/2, Selector2/2, Selector5/2, Selector4/2  "i=1:N"
  Omega/1 -> Selector2/1
  number of  iterations/1 -> For Iterator/1
  Sum4/1 -> Memory2/1, tau_WF/1
  Memory2/1 -> Sum4/2
  Product1/1 -> Sum4/1
  Selector5/1 -> Sum5/2  "phase"
  Selector3/1 -> "[-inf inf] to [-pi pi]"/1  "psi_r"
  "                "/1 -> Product1/1
  Product4/1 -> Product1/2
  one/1 -> Sum2/1
  Sum2/1 -> Force RAO tables/1(beta_idx), WD RAO tables/1(beta_idx)
  Prelookup/1 -> Sum2/2
  Abs/1 -> Prelookup/1
  Sign/1 -> Force RAO tables/2(sign), WD RAO tables/2(sign)
  Sum1/1 -> Memory1/1, tau_WD/1
  Memory1/1 -> Sum1/2
  Product3/1 -> Sum1/1
  WD RAO tables/1(amp) -> Product3/1
  "[-inf inf] to [-pi pi]"/1 -> Abs/1, Sign/1
  Prelookup1/1 -> Sum6/1
  one1/1 -> Sum3/2, Sum6/2
  Sum3/1 -> Mux/2
  Sum6/1 -> Sum3/1, Mux/1
  Selector2/1 -> Prelookup1/1  "omega"
  Mux/1 -> Force RAO tables/3(w_idx_12), WD RAO tables/3(w_idx_12)  "w_idx_12"
  Prelookup1/2 -> Force RAO tables/4(f), WD RAO tables/4(f)  "f"

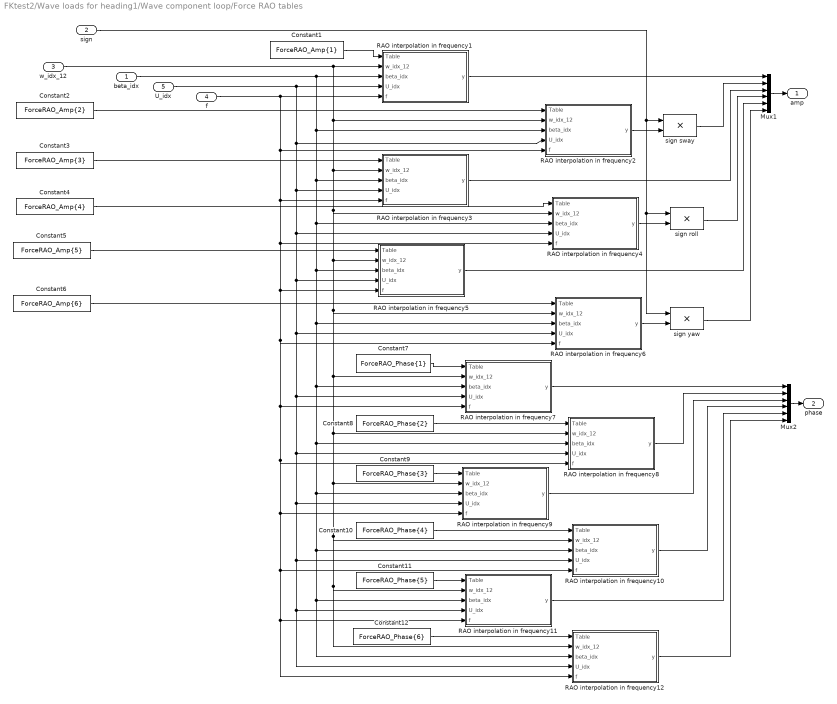
== system FKtest2/Wave loads for heading1/Wave component loop/Force RAO tables ==
  beta_idx : Inport
  sign : Inport  Port=2
  w_idx_12 : Inport  Port=3
  f : Inport  Port=4
  U_idx : Inport  Port=5
  Constant1 : Constant  Value=ForceRAO_Amp{1}
  Constant10 : Constant  Value=ForceRAO_Phase{4}
  Constant11 : Constant  Value=ForceRAO_Phase{5}
  Constant12 : Constant  Value=ForceRAO_Phase{6}
  Constant2 : Constant  Value=ForceRAO_Amp{2}
  Constant3 : Constant  Value=ForceRAO_Amp{3}
  Constant4 : Constant  Value=ForceRAO_Amp{4}
  Constant5 : Constant  Value=ForceRAO_Amp{5}
  Constant6 : Constant  Value=ForceRAO_Amp{6}
  Constant7 : Constant  Value=ForceRAO_Phase{1}
  Constant8 : Constant  Value=ForceRAO_Phase{2}
  Constant9 : Constant  Value=ForceRAO_Phase{3}
  Mux1 : Mux  Inputs=6
  Mux2 : Mux  Inputs=6
  RAO interpolation in frequency1 : Subsystem
  RAO interpolation in frequency10 : Subsystem
  RAO interpolation in frequency11 : Subsystem
  RAO interpolation in frequency12 : Subsystem
  RAO interpolation in frequency2 : Subsystem
  RAO interpolation in frequency3 : Subsystem
  RAO interpolation in frequency4 : Subsystem
  RAO interpolation in frequency5 : Subsystem
  RAO interpolation in frequency6 : Subsystem
  RAO interpolation in frequency7 : Subsystem
  RAO interpolation in frequency8 : Subsystem
  RAO interpolation in frequency9 : Subsystem
  sign roll : Product  Inputs=**  SaturateOnIntegerOverflow=on
  sign sway : Product  Inputs=**  SaturateOnIntegerOverflow=on
  sign yaw : Product  Inputs=**  SaturateOnIntegerOverflow=on
  amp : Outport
  phase : Outport  Port=2
  wires:
  Mux1/1 -> amp/1
  Mux2/1 -> phase/1
  sign/1 -> sign yaw/1, sign roll/1, sign sway/1
  RAO interpolation in frequency6/1(y) -> sign yaw/2
  sign yaw/1 -> Mux1/6
  sign roll/1 -> Mux1/4
  RAO interpolation in frequency2/1(y) -> sign sway/2
  sign sway/1 -> Mux1/2
  RAO interpolation in frequency5/1(y) -> Mux1/5
  RAO interpolation in frequency3/1(y) -> Mux1/3
  RAO interpolation in frequency1/1(y) -> Mux1/1
  Constant1/1 -> RAO interpolation in frequency1/1(Table)
  Constant2/1 -> RAO interpolation in frequency2/1(Table)
  Constant3/1 -> RAO interpolation in frequency3/1(Table)
  U_idx/1 -> RAO interpolation in frequency1/4(U_idx), RAO interpolation in frequency11/4(U_idx), RAO interpolation in frequency12/4(U_idx), RAO interpolation in frequency10/4(U_idx), RAO interpolation in frequency9/4(U_idx), RAO interpolation in frequency8/4(U_idx), RAO interpolation in frequency7/4(U_idx), RAO interpolation in frequency6/4(U_idx), RAO interpolation in frequency5/4(U_idx), RAO interpolation in frequency4/4(U_idx), RAO interpolation in frequency3/4(U_idx), RAO interpolation in frequency2/4(U_idx)
  Constant4/1 -> RAO interpolation in frequency4/1(Table)
  RAO interpolation in frequency4/1(y) -> sign roll/2
  Constant5/1 -> RAO interpolation in frequency5/1(Table)
  Constant6/1 -> RAO interpolation in frequency6/1(Table)
  RAO interpolation in frequency12/1(y) -> Mux2/6
  RAO interpolation in frequency8/1(y) -> Mux2/2
  Constant8/1 -> RAO interpolation in frequency8/1(Table)
  Constant9/1 -> RAO interpolation in frequency9/1(Table)
  Constant10/1 -> RAO interpolation in frequency10/1(Table)
  RAO interpolation in frequency10/1(y) -> Mux2/4
  Constant11/1 -> RAO interpolation in frequency11/1(Table)
  Constant12/1 -> RAO interpolation in frequency12/1(Table)
  beta_idx/1 -> RAO interpolation in frequency11/3(beta_idx), RAO interpolation in frequency12/3(beta_idx), RAO interpolation in frequency10/3(beta_idx), RAO interpolation in frequency9/3(beta_idx), RAO interpolation in frequency8/3(beta_idx), RAO interpolation in frequency7/3(beta_idx), RAO interpolation in frequency6/3(beta_idx), RAO interpolation in frequency5/3(beta_idx), RAO interpolation in frequency4/3(beta_idx), RAO interpolation in frequency3/3(beta_idx), RAO interpolation in frequency2/3(beta_idx), RAO interpolation in frequency1/3(beta_idx)
  RAO interpolation in frequency7/1(y) -> Mux2/1
  RAO interpolation in frequency9/1(y) -> Mux2/3
  RAO interpolation in frequency11/1(y) -> Mux2/5
  w_idx_12/1 -> RAO interpolation in frequency1/2(w_idx_12), RAO interpolation in frequency2/2(w_idx_12), RAO interpolation in frequency3/2(w_idx_12), RAO interpolation in frequency4/2(w_idx_12), RAO interpolation in frequency5/2(w_idx_12), RAO interpolation in frequency6/2(w_idx_12), RAO interpolation in frequency7/2(w_idx_12), RAO interpolation in frequency8/2(w_idx_12), RAO interpolation in frequency9/2(w_idx_12), RAO interpolation in frequency10/2(w_idx_12), RAO interpolation in frequency11/2(w_idx_12), RAO interpolation in frequency12/2(w_idx_12)
  f/1 -> RAO interpolation in frequency1/5(f), RAO interpolation in frequency2/5(f), RAO interpolation in frequency3/5(f), RAO interpolation in frequency4/5(f), RAO interpolation in frequency5/5(f), RAO interpolation in frequency6/5(f), RAO interpolation in frequency7/5(f), RAO interpolation in frequency8/5(f), RAO interpolation in frequency9/5(f), RAO interpolation in frequency10/5(f), RAO interpolation in frequency11/5(f), RAO interpolation in frequency12/5(f)
  Constant7/1 -> RAO interpolation in frequency7/1(Table)

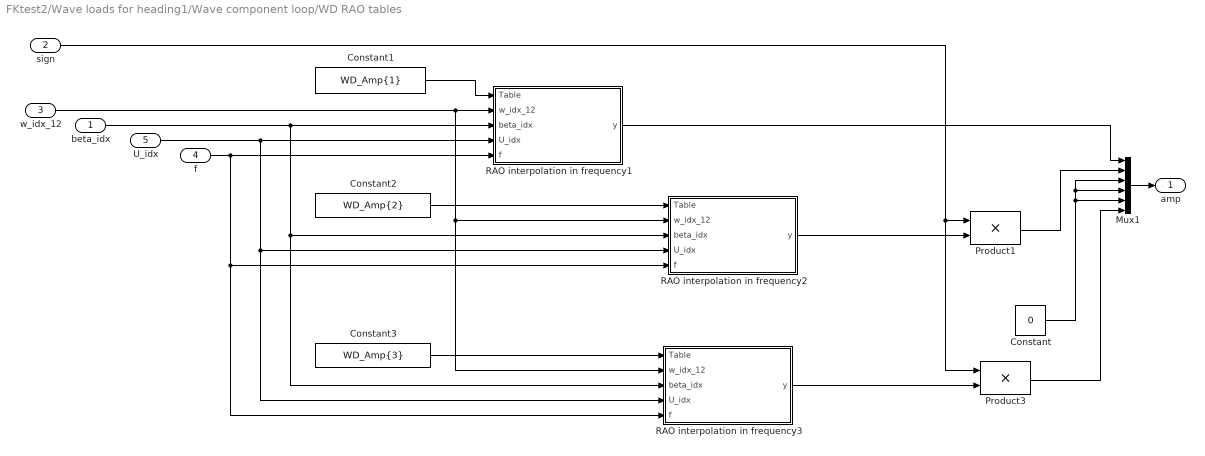
== system FKtest2/Wave loads for heading1/Wave component loop/WD RAO tables ==
  beta_idx : Inport
  sign : Inport  Port=2
  w_idx_12 : Inport  Port=3
  f : Inport  Port=4
  U_idx : Inport  Port=5
  Constant : Constant  Value=0
  Constant1 : Constant  Value=WD_Amp{1}
  Constant2 : Constant  Value=WD_Amp{2}
  Constant3 : Constant  Value=WD_Amp{3}
  Mux1 : Mux  Inputs=6
  Product1 : Product  Inputs=**  SaturateOnIntegerOverflow=on
  Product3 : Product  Inputs=**  SaturateOnIntegerOverflow=on
  RAO interpolation in frequency1 : Subsystem
  RAO interpolation in frequency2 : Subsystem
  RAO interpolation in frequency3 : Subsystem
  amp : Outport
  wires:
  Mux1/1 -> amp/1
  sign/1 -> Product1/1, Product3/1
  RAO interpolation in frequency3/1(y) -> Product3/2
  Product3/1 -> Mux1/6
  RAO interpolation in frequency2/1(y) -> Product1/2
  Product1/1 -> Mux1/2
  RAO interpolation in frequency1/1(y) -> Mux1/1
  Constant1/1 -> RAO interpolation in frequency1/1(Table)
  Constant2/1 -> RAO interpolation in frequency2/1(Table)
  U_idx/1 -> RAO interpolation in frequency2/4(U_idx), RAO interpolation in frequency3/4(U_idx), RAO interpolation in frequency1/4(U_idx)
  Constant3/1 -> RAO interpolation in frequency3/1(Table)
  beta_idx/1 -> RAO interpolation in frequency2/3(beta_idx), RAO interpolation in frequency3/3(beta_idx), RAO interpolation in frequency1/3(beta_idx)
  Constant/1 -> Mux1/3, Mux1/4, Mux1/5
  w_idx_12/1 -> RAO interpolation in frequency1/2(w_idx_12), RAO interpolation in frequency2/2(w_idx_12), RAO interpolation in frequency3/2(w_idx_12)
  f/1 -> RAO interpolation in frequency1/5(f), RAO interpolation in frequency2/5(f), RAO interpolation in frequency3/5(f)
